simulink model "MultiLoop_mode3"  (Simulink 10.0)
settings: Solver=ode45  StartTime=0.0  StopTime=72  FixedStep=Ts_base  MinStep=1e-6  RelTol=1e-6
values from neighbouring files (symbols this model uses):
  xInitial = xFinal    [prepNextSimIteration.m]
undefined symbols (not defined in the file or in its folder): IDV_Init, r1_0, r4_0, seed, Ts_base, Ts_save
undefined symbols (not defined in the file): SetPoint_Init, SP_deltaTRamp
libraries: TElib x17, simulink x12
settings Model: Creator=ricker  LastModifiedBy=christopher
settings DataIOCC: LoadInitialState=on  SaveFinalState=on  SaveFormat=Structure  SignalLoggingSaveFormat=ModelDataLogs  SaveOutput=off  SaveTime=off  SignalLoggingName=sigsOut
settings OptimizationCC: InitFltsAndDblsToZero=on
settings DebuggingCC: SaveWithParameterizedLinksMsg=none  SignalResolutionControl=TryResolveAllWithWarning  MultiTaskDSMMsg=warning  MultiTaskCondExecSysMsg=none  FcnCallInpInsideContextMsg=warning
settings HardwareCC: TargetUnknown=on
settings GRTTargetCC: TargetFcnLib=ansi_tfl_tmw.mat  GeneratePreprocessorConditionals=Disable all
settings ConfigComp: CovExternalEMLEnable=off  CovSFcnEnable=off

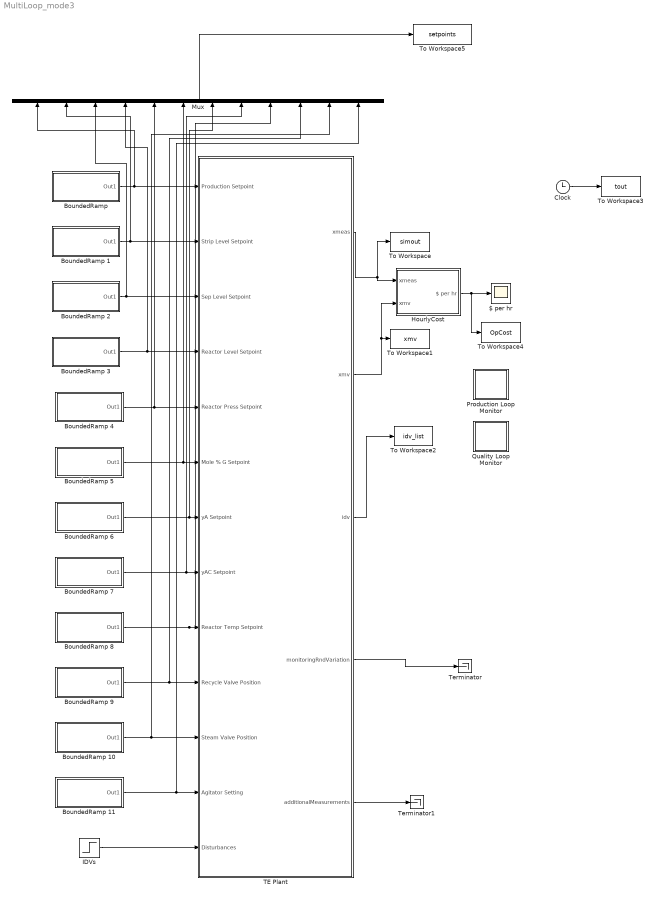
== system MultiLoop_mode3 ==
  $ per hr : Scope
  "BoundedRamp " : Subsystem  mask{SP_before=SetPoint_Init(1,1), SP_after=SetPoint_Init(2,1), tRampStart=SetPoint_Init(3,1), deltaT_ramp=SP_deltaTRamp}
      mask prompts: SP_before "Value before ramp"; SP_after "Value after ramp"; tRampStart "Ramp start time"; deltaT_ramp "Ramp transition time"
  BoundedRamp 1 : Subsystem  mask{SP_before=SetPoint_Init(1,2), SP_after=SetPoint_Init(2,2), tRampStart=SetPoint_Init(3,2), deltaT_ramp=SP_deltaTRamp}
      mask prompts: SP_before "Value before ramp"; SP_after "Value after ramp"; tRampStart "Ramp start time"; deltaT_ramp "Ramp transition time"
  BoundedRamp 10 : Subsystem  mask{SP_before=SetPoint_Init(1,11), SP_after=SetPoint_Init(2,11), tRampStart=SetPoint_Init(3,11), deltaT_ramp=SP_deltaTRamp}
      mask prompts: SP_before "Value before ramp"; SP_after "Value after ramp"; tRampStart "Ramp start time"; deltaT_ramp "Ramp transition time"
  BoundedRamp 11 : Subsystem  mask{SP_before=SetPoint_Init(1,12), SP_after=SetPoint_Init(2,12), tRampStart=SetPoint_Init(3,12), deltaT_ramp=SP_deltaTRamp}
      mask prompts: SP_before "Value before ramp"; SP_after "Value after ramp"; tRampStart "Ramp start time"; deltaT_ramp "Ramp transition time"
  BoundedRamp 2 : Subsystem  mask{SP_before=SetPoint_Init(1,3), SP_after=SetPoint_Init(2,3), tRampStart=SetPoint_Init(3,3), deltaT_ramp=SP_deltaTRamp}
      mask prompts: SP_before "Value before ramp"; SP_after "Value after ramp"; tRampStart "Ramp start time"; deltaT_ramp "Ramp transition time"
  BoundedRamp 3 : Subsystem  mask{SP_before=SetPoint_Init(1,4), SP_after=SetPoint_Init(2,4), tRampStart=SetPoint_Init(3,4), deltaT_ramp=SP_deltaTRamp}
      mask prompts: SP_before "Value before ramp"; SP_after "Value after ramp"; tRampStart "Ramp start time"; deltaT_ramp "Ramp transition time"
  BoundedRamp 4 : Subsystem  mask{SP_before=SetPoint_Init(1,5), SP_after=SetPoint_Init(2,5), tRampStart=SetPoint_Init(3,5), deltaT_ramp=SP_deltaTRamp}
      mask prompts: SP_before "Value before ramp"; SP_after "Value after ramp"; tRampStart "Ramp start time"; deltaT_ramp "Ramp transition time"
  BoundedRamp 5 : Subsystem  mask{SP_before=SetPoint_Init(1,6), SP_after=SetPoint_Init(2,6), tRampStart=SetPoint_Init(3,6), deltaT_ramp=SP_deltaTRamp}
      mask prompts: SP_before "Value before ramp"; SP_after "Value after ramp"; tRampStart "Ramp start time"; deltaT_ramp "Ramp transition time"
  BoundedRamp 6 : Subsystem  mask{SP_before=SetPoint_Init(1,7), SP_after=SetPoint_Init(2,7), tRampStart=SetPoint_Init(3,7), deltaT_ramp=SP_deltaTRamp}
      mask prompts: SP_before "Value before ramp"; SP_after "Value after ramp"; tRampStart "Ramp start time"; deltaT_ramp "Ramp transition time"
  BoundedRamp 7 : Subsystem  mask{SP_before=SetPoint_Init(1,8), SP_after=SetPoint_Init(2,8), tRampStart=SetPoint_Init(3,8), deltaT_ramp=SP_deltaTRamp}
      mask prompts: SP_before "Value before ramp"; SP_after "Value after ramp"; tRampStart "Ramp start time"; deltaT_ramp "Ramp transition time"
  BoundedRamp 8 : Subsystem  mask{SP_before=SetPoint_Init(1,9), SP_after=SetPoint_Init(2,9), tRampStart=SetPoint_Init(3,9), deltaT_ramp=SP_deltaTRamp}
      mask prompts: SP_before "Value before ramp"; SP_after "Value after ramp"; tRampStart "Ramp start time"; deltaT_ramp "Ramp transition time"
  BoundedRamp 9 : Subsystem  mask{SP_before=SetPoint_Init(1,10), SP_after=SetPoint_Init(2,10), tRampStart=SetPoint_Init(3,10), deltaT_ramp=SP_deltaTRamp}
      mask prompts: SP_before "Value before ramp"; SP_after "Value after ramp"; tRampStart "Ramp start time"; deltaT_ramp "Ramp transition time"
  Clock : Clock
  HourlyCost : Subsystem
  IDVs : Step  Time=IDV_Init(3,:)  Before=IDV_Init(1,:)  After=IDV_Init(2,:)  SampleTime=0
  Mux : Mux  Inputs=12
  Production Loop Monitor : Subsystem
  Quality Loop Monitor : Subsystem
  TE Plant : Subsystem
  Terminator : Terminator
  Terminator1 : Terminator
  To Workspace : ToWorkspace  VariableName=simout  SampleTime=Ts_save
  To Workspace1 : ToWorkspace  VariableName=xmv  SampleTime=Ts_save
  To Workspace2 : ToWorkspace  VariableName=idv_list  SampleTime=Ts_save
  To Workspace3 : ToWorkspace  VariableName=tout  SampleTime=Ts_save
  To Workspace4 : ToWorkspace  VariableName=OpCost  SampleTime=Ts_save
  To Workspace5 : ToWorkspace  VariableName=setpoints  SampleTime=Ts_save
  wires:
  TE Plant/1(xmeas) -> HourlyCost/1(xmeas), To Workspace/1
  TE Plant/2(xmv) -> To Workspace1/1, HourlyCost/2(xmv)
  TE Plant/3(idv) -> To Workspace2/1
  Clock/1 -> To Workspace3/1
  HourlyCost/1($ per hr) -> $ per hr/1, To Workspace4/1
  "BoundedRamp "/1(Out1) -> TE Plant/1(Production Setpoint), Mux/1
  BoundedRamp 11/1(Out1) -> Mux/12, TE Plant/12(Agitator Setting)
  BoundedRamp 10/1(Out1) -> Mux/11, TE Plant/11(Steam Valve Position)
  BoundedRamp 9/1(Out1) -> Mux/10, TE Plant/10(Recycle Valve Position)
  BoundedRamp 8/1(Out1) -> Mux/9, TE Plant/9(Reactor Temp Setpoint)
  BoundedRamp 7/1(Out1) -> Mux/8, TE Plant/8(yAC Setpoint)
  BoundedRamp 6/1(Out1) -> Mux/7, TE Plant/7(yA Setpoint)
  BoundedRamp 5/1(Out1) -> Mux/6, TE Plant/6(Mole % G Setpoint)
  BoundedRamp 4/1(Out1) -> TE Plant/5(Reactor Press Setpoint), Mux/5
  BoundedRamp 3/1(Out1) -> TE Plant/4(Reactor Level Setpoint), Mux/4
  BoundedRamp 2/1(Out1) -> TE Plant/3(Sep Level Setpoint), Mux/3
  BoundedRamp 1/1(Out1) -> TE Plant/2(Strip Level Setpoint), Mux/2
  IDVs/1 -> TE Plant/13(Disturbances)
  Mux/1 -> To Workspace5/1
  TE Plant/4(monitoringRndVariation) -> Terminator/1
  TE Plant/5(additionalMeasurements) -> Terminator1/1

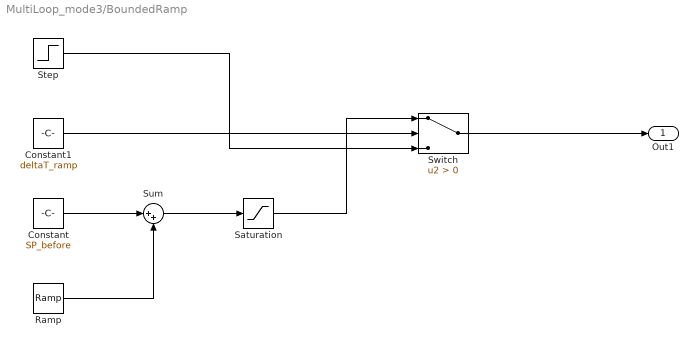
== system MultiLoop_mode3/BoundedRamp  ==
  Constant : Constant  Value=SP_before
  Constant1 : Constant  Value=deltaT_ramp
  Ramp : simulink/Sources/Ramp  slope=(SP_after-SP_before) /max(deltaT_ramp,0.1)  start=tRampStart  InitialOutput=0
  Saturation : Saturate  UpperLimit=max(SP_before, SP_after)  LowerLimit=min(SP_before, SP_after)
  Step : Step  Time=tRampStart  Before=SP_before  After=SP_after  SampleTime=0
  Sum : Sum  Inputs=|++
  Switch : Switch  Criteria=u2 > Threshold
  Out1 : Outport  VectorParamsAs1DForOutWhenUnconnected=off
  wires:
  Constant/1 -> Sum/1
  Ramp/1 -> Sum/2
  Sum/1 -> Saturation/1
  Constant1/1 -> Switch/2
  Switch/1 -> Out1/1
  Step/1 -> Switch/3
  Saturation/1 -> Switch/1

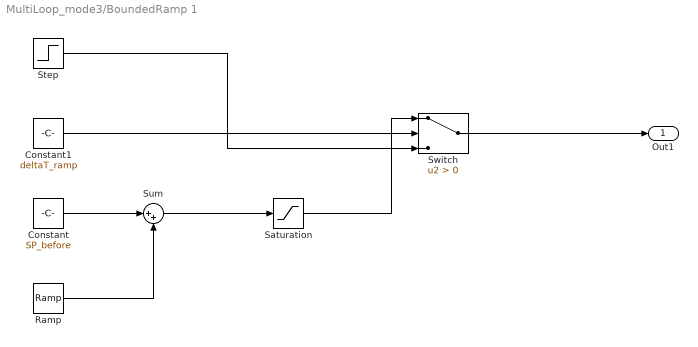
== system MultiLoop_mode3/BoundedRamp 1 ==
  Constant : Constant  Value=SP_before
  Constant1 : Constant  Value=deltaT_ramp
  Ramp : simulink/Sources/Ramp  slope=(SP_after-SP_before) /max(deltaT_ramp,0.1)  start=tRampStart  InitialOutput=0
  Saturation : Saturate  UpperLimit=max(SP_before, SP_after)  LowerLimit=min(SP_before, SP_after)
  Step : Step  Time=tRampStart  Before=SP_before  After=SP_after  SampleTime=0
  Sum : Sum  Inputs=|++
  Switch : Switch  Criteria=u2 > Threshold
  Out1 : Outport  VectorParamsAs1DForOutWhenUnconnected=off
  wires:
  Constant/1 -> Sum/1
  Ramp/1 -> Sum/2
  Sum/1 -> Saturation/1
  Constant1/1 -> Switch/2
  Switch/1 -> Out1/1
  Step/1 -> Switch/3
  Saturation/1 -> Switch/1

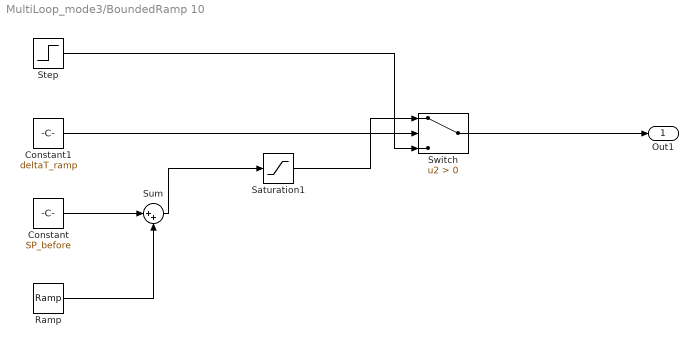
== system MultiLoop_mode3/BoundedRamp 10 ==
  Constant : Constant  Value=SP_before
  Constant1 : Constant  Value=deltaT_ramp
  Ramp : simulink/Sources/Ramp  slope=(SP_after-SP_before) /max(deltaT_ramp,0.1)  start=tRampStart  InitialOutput=0
  Saturation1 : Saturate  UpperLimit=max(SP_before, SP_after)  LowerLimit=min(SP_before, SP_after)
  Step : Step  Time=tRampStart  Before=SP_before  After=SP_after  SampleTime=0
  Sum : Sum  Inputs=|++
  Switch : Switch  Criteria=u2 > Threshold
  Out1 : Outport  VectorParamsAs1DForOutWhenUnconnected=off
  wires:
  Constant/1 -> Sum/1
  Ramp/1 -> Sum/2
  Sum/1 -> Saturation1/1
  Constant1/1 -> Switch/2
  Switch/1 -> Out1/1
  Step/1 -> Switch/3
  Saturation1/1 -> Switch/1

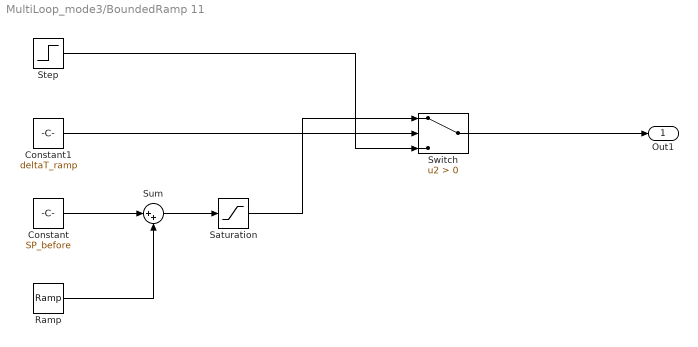
== system MultiLoop_mode3/BoundedRamp 11 ==
  Constant : Constant  Value=SP_before
  Constant1 : Constant  Value=deltaT_ramp
  Ramp : simulink/Sources/Ramp  slope=(SP_after-SP_before) /max(deltaT_ramp,0.1)  start=tRampStart  InitialOutput=0
  Saturation : Saturate  UpperLimit=max(SP_before, SP_after)  LowerLimit=min(SP_before, SP_after)
  Step : Step  Time=tRampStart  Before=SP_before  After=SP_after  SampleTime=0
  Sum : Sum  Inputs=|++
  Switch : Switch  Criteria=u2 > Threshold
  Out1 : Outport  VectorParamsAs1DForOutWhenUnconnected=off
  wires:
  Constant/1 -> Sum/1
  Ramp/1 -> Sum/2
  Sum/1 -> Saturation/1
  Constant1/1 -> Switch/2
  Switch/1 -> Out1/1
  Step/1 -> Switch/3
  Saturation/1 -> Switch/1

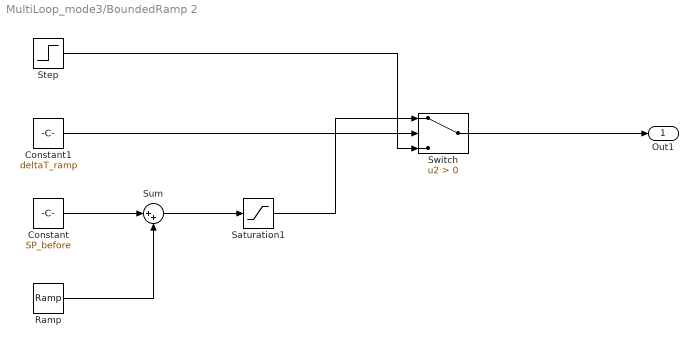
== system MultiLoop_mode3/BoundedRamp 2 ==
  Constant : Constant  Value=SP_before
  Constant1 : Constant  Value=deltaT_ramp
  Ramp : simulink/Sources/Ramp  slope=(SP_after-SP_before) /max(deltaT_ramp,0.1)  start=tRampStart  InitialOutput=0
  Saturation1 : Saturate  UpperLimit=max(SP_before, SP_after)  LowerLimit=min(SP_before, SP_after)
  Step : Step  Time=tRampStart  Before=SP_before  After=SP_after  SampleTime=0
  Sum : Sum  Inputs=|++
  Switch : Switch  Criteria=u2 > Threshold
  Out1 : Outport  VectorParamsAs1DForOutWhenUnconnected=off
  wires:
  Constant/1 -> Sum/1
  Ramp/1 -> Sum/2
  Sum/1 -> Saturation1/1
  Constant1/1 -> Switch/2
  Switch/1 -> Out1/1
  Step/1 -> Switch/3
  Saturation1/1 -> Switch/1

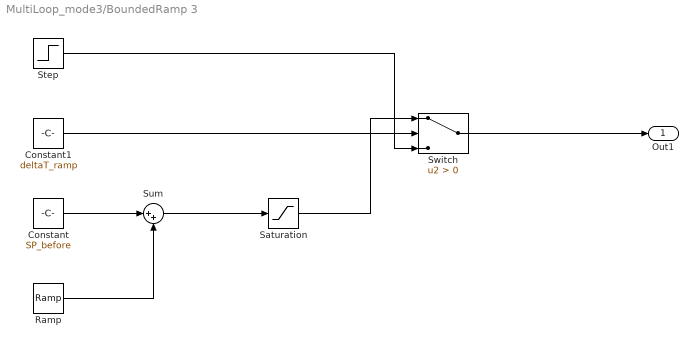
== system MultiLoop_mode3/BoundedRamp 3 ==
  Constant : Constant  Value=SP_before
  Constant1 : Constant  Value=deltaT_ramp
  Ramp : simulink/Sources/Ramp  slope=(SP_after-SP_before) /max(deltaT_ramp,0.1)  start=tRampStart  InitialOutput=0
  Saturation : Saturate  UpperLimit=max(SP_before, SP_after)  LowerLimit=min(SP_before, SP_after)
  Step : Step  Time=tRampStart  Before=SP_before  After=SP_after  SampleTime=0
  Sum : Sum  Inputs=|++
  Switch : Switch  Criteria=u2 > Threshold
  Out1 : Outport  VectorParamsAs1DForOutWhenUnconnected=off
  wires:
  Constant/1 -> Sum/1
  Ramp/1 -> Sum/2
  Sum/1 -> Saturation/1
  Constant1/1 -> Switch/2
  Switch/1 -> Out1/1
  Step/1 -> Switch/3
  Saturation/1 -> Switch/1

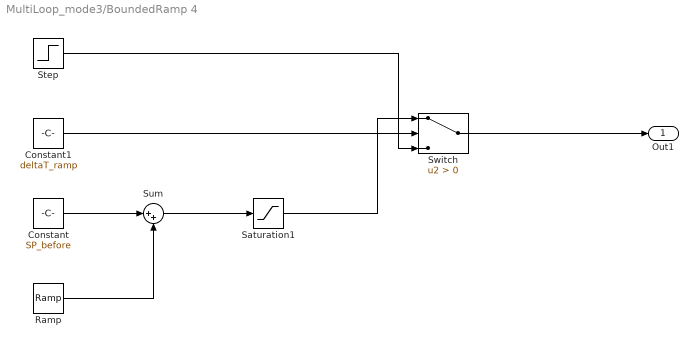
== system MultiLoop_mode3/BoundedRamp 4 ==
  Constant : Constant  Value=SP_before
  Constant1 : Constant  Value=deltaT_ramp
  Ramp : simulink/Sources/Ramp  slope=(SP_after-SP_before) /max(deltaT_ramp,0.1)  start=tRampStart  InitialOutput=0
  Saturation1 : Saturate  UpperLimit=max(SP_before, SP_after)  LowerLimit=min(SP_before, SP_after)
  Step : Step  Time=tRampStart  Before=SP_before  After=SP_after  SampleTime=0
  Sum : Sum  Inputs=|++
  Switch : Switch  Criteria=u2 > Threshold
  Out1 : Outport  VectorParamsAs1DForOutWhenUnconnected=off
  wires:
  Constant/1 -> Sum/1
  Ramp/1 -> Sum/2
  Sum/1 -> Saturation1/1
  Constant1/1 -> Switch/2
  Switch/1 -> Out1/1
  Step/1 -> Switch/3
  Saturation1/1 -> Switch/1

== system MultiLoop_mode3/BoundedRamp 5 ==
  Constant : Constant  Value=SP_before
  Constant1 : Constant  Value=deltaT_ramp
  Ramp : simulink/Sources/Ramp  slope=(SP_after-SP_before) /max(deltaT_ramp,0.1)  start=tRampStart  InitialOutput=0
  Saturation1 : Saturate  UpperLimit=max(SP_before, SP_after)  LowerLimit=min(SP_before, SP_after)
  Step : Step  Time=tRampStart  Before=SP_before  After=SP_after  SampleTime=0
  Sum : Sum  Inputs=|++
  Switch : Switch  Criteria=u2 > Threshold
  Out1 : Outport  VectorParamsAs1DForOutWhenUnconnected=off
  wires:
  Constant/1 -> Sum/1
  Ramp/1 -> Sum/2
  Sum/1 -> Saturation1/1
  Constant1/1 -> Switch/2
  Switch/1 -> Out1/1
  Step/1 -> Switch/3
  Saturation1/1 -> Switch/1

== system MultiLoop_mode3/BoundedRamp 6 ==
  Constant : Constant  Value=SP_before
  Constant1 : Constant  Value=deltaT_ramp
  Ramp : simulink/Sources/Ramp  slope=(SP_after-SP_before) /max(deltaT_ramp,0.1)  start=tRampStart  InitialOutput=0
  Saturation1 : Saturate  UpperLimit=max(SP_before, SP_after)  LowerLimit=min(SP_before, SP_after)
  Step : Step  Time=tRampStart  Before=SP_before  After=SP_after  SampleTime=0
  Sum : Sum  Inputs=|++
  Switch : Switch  Criteria=u2 > Threshold
  Out1 : Outport  VectorParamsAs1DForOutWhenUnconnected=off
  wires:
  Constant/1 -> Sum/1
  Ramp/1 -> Sum/2
  Sum/1 -> Saturation1/1
  Constant1/1 -> Switch/2
  Switch/1 -> Out1/1
  Step/1 -> Switch/3
  Saturation1/1 -> Switch/1

== system MultiLoop_mode3/BoundedRamp 7 ==
  Constant : Constant  Value=SP_before
  Constant1 : Constant  Value=deltaT_ramp
  Ramp : simulink/Sources/Ramp  slope=(SP_after-SP_before) /max(deltaT_ramp,0.1)  start=tRampStart  InitialOutput=0
  Saturation1 : Saturate  UpperLimit=max(SP_before, SP_after)  LowerLimit=min(SP_before, SP_after)
  Step : Step  Time=tRampStart  Before=SP_before  After=SP_after  SampleTime=0
  Sum : Sum  Inputs=|++
  Switch : Switch  Criteria=u2 > Threshold
  Out1 : Outport  VectorParamsAs1DForOutWhenUnconnected=off
  wires:
  Constant/1 -> Sum/1
  Ramp/1 -> Sum/2
  Sum/1 -> Saturation1/1
  Constant1/1 -> Switch/2
  Switch/1 -> Out1/1
  Step/1 -> Switch/3
  Saturation1/1 -> Switch/1

== system MultiLoop_mode3/BoundedRamp 8 ==
  Constant : Constant  Value=SP_before
  Constant1 : Constant  Value=deltaT_ramp
  Ramp : simulink/Sources/Ramp  slope=(SP_after-SP_before) /max(deltaT_ramp,0.1)  start=tRampStart  InitialOutput=0
  Saturation1 : Saturate  UpperLimit=max(SP_before, SP_after)  LowerLimit=min(SP_before, SP_after)
  Step : Step  Time=tRampStart  Before=SP_before  After=SP_after  SampleTime=0
  Sum : Sum  Inputs=|++
  Switch : Switch  Criteria=u2 > Threshold
  Out1 : Outport  VectorParamsAs1DForOutWhenUnconnected=off
  wires:
  Constant/1 -> Sum/1
  Ramp/1 -> Sum/2
  Sum/1 -> Saturation1/1
  Constant1/1 -> Switch/2
  Switch/1 -> Out1/1
  Step/1 -> Switch/3
  Saturation1/1 -> Switch/1

== system MultiLoop_mode3/BoundedRamp 9 ==
  Constant : Constant  Value=SP_before
  Constant1 : Constant  Value=deltaT_ramp
  Ramp : simulink/Sources/Ramp  slope=(SP_after-SP_before) /max(deltaT_ramp,0.1)  start=tRampStart  InitialOutput=0
  Saturation1 : Saturate  UpperLimit=max(SP_before, SP_after)  LowerLimit=min(SP_before, SP_after)
  Step : Step  Time=tRampStart  Before=SP_before  After=SP_after  SampleTime=0
  Sum : Sum  Inputs=|++
  Switch : Switch  Criteria=u2 > Threshold
  Out1 : Outport  VectorParamsAs1DForOutWhenUnconnected=off
  wires:
  Constant/1 -> Sum/1
  Ramp/1 -> Sum/2
  Sum/1 -> Saturation1/1
  Constant1/1 -> Switch/2
  Switch/1 -> Out1/1
  Step/1 -> Switch/3
  Saturation1/1 -> Switch/1

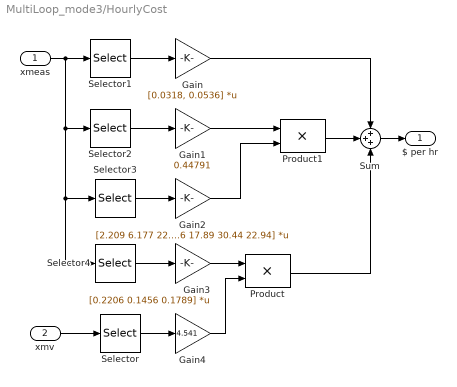
== system MultiLoop_mode3/HourlyCost ==
  xmeas : Inport  PortDimensions=41
  xmv : Inport  Port=2  PortDimensions=12
  Gain : Gain  Gain=[0.0318, 0.0536]  Multiplication=Matrix(K*u)  SaturateOnIntegerOverflow=on  OutDataTypeStr=Inherit: Same as input  ParamDataTypeStr=Inherit: Same as input
  Gain1 : Gain  Gain=0.44791  SaturateOnIntegerOverflow=on  OutDataTypeStr=Inherit: Same as input  ParamDataTypeStr=Inherit: Same as input
  Gain2 : Gain  Gain=[2.209 6.177 22.06 14.56 17.89 30.44 22.94]  Multiplication=Matrix(K*u)  SaturateOnIntegerOverflow=on  OutDataTypeStr=Inherit: Same as input  ParamDataTypeStr=Inherit: Same as input
  Gain3 : Gain  Gain=[0.2206 0.1456 0.1789]  Multiplication=Matrix(K*u)  SaturateOnIntegerOverflow=on  OutDataTypeStr=Inherit: Same as input  ParamDataTypeStr=Inherit: Same as input
  Gain4 : Gain  Gain=4.541  SaturateOnIntegerOverflow=on  OutDataTypeStr=Inherit: Same as input  ParamDataTypeStr=Inherit: Same as input
  Product : Product  SaturateOnIntegerOverflow=on  OutDataTypeStr=Inherit: Same as first input
  Product1 : Product  SaturateOnIntegerOverflow=on  OutDataTypeStr=Inherit: Same as first input
  Selector : Selector  InputPortWidth=12  IndexOptions=Index vector (dialog)  Indices=8  OutputSizes=1
  Selector1 : Selector  InputPortWidth=41  IndexOptions=Index vector (dialog)  Indices=[19 20]  OutputSizes=1
  Selector2 : Selector  InputPortWidth=41  IndexOptions=Index vector (dialog)  Indices=[10]  OutputSizes=1
  Selector3 : Selector  InputPortWidth=41  IndexOptions=Index vector (dialog)  Indices=[29, 31:36]  OutputSizes=1
  Selector4 : Selector  InputPortWidth=41  IndexOptions=Index vector (dialog)  Indices=[37:39]  OutputSizes=1
  Sum : Sum  Inputs=+++  SaturateOnIntegerOverflow=on
  $ per hr : Outport  VectorParamsAs1DForOutWhenUnconnected=off
  wires:
  xmv/1 -> Selector/1
  xmeas/1 -> Selector1/1, Selector2/1, Selector3/1, Selector4/1
  Selector1/1 -> Gain/1
  Selector2/1 -> Gain1/1
  Selector3/1 -> Gain2/1
  Selector4/1 -> Gain3/1
  Selector/1 -> Gain4/1
  Gain3/1 -> Product/1
  Gain4/1 -> Product/2
  Sum/1 -> $ per hr/1
  Product/1 -> Sum/3
  Gain/1 -> Sum/1
  Product1/1 -> Sum/2
  Gain1/1 -> Product1/1
  Gain2/1 -> Product1/2

== system MultiLoop_mode3/Production Loop Monitor ==
  Mux2 : Mux  Inputs=2
  Production : Scope
  wires:
  Mux2/1 -> Production/1
  [xmeas17] -> Mux2/2
  [Prodsp] -> Mux2/1

== system MultiLoop_mode3/Quality Loop Monitor ==
  Mux2 : Mux  Inputs=2
  Quality : Scope
  wires:
  [PctGsp] -> Mux2/1
  [xmeas40] -> Mux2/2
  Mux2/1 -> Quality/1

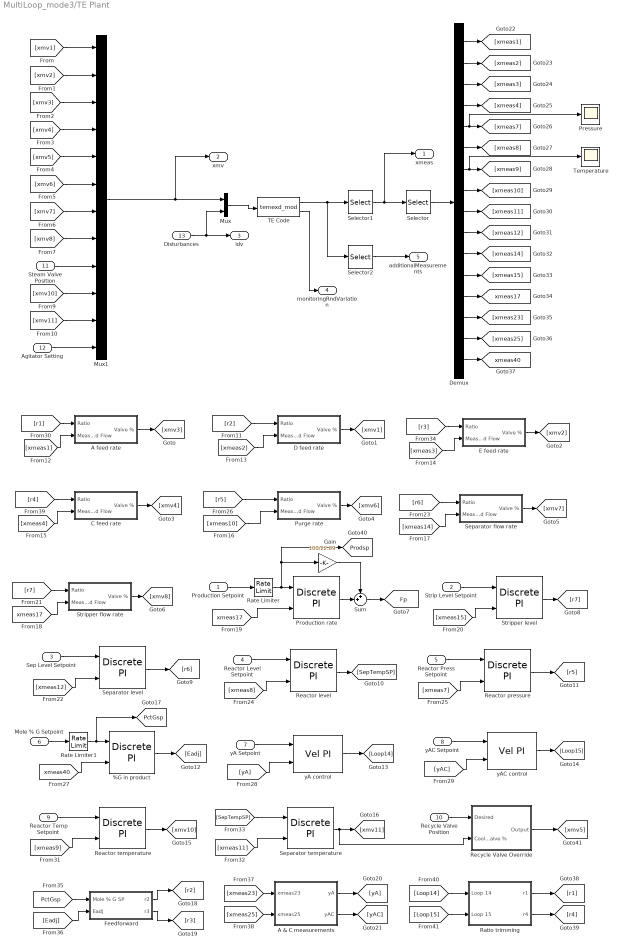
== system MultiLoop_mode3/TE Plant ==
  Production Setpoint : Inport
  Strip Level Setpoint : Inport  Port=2
  Sep Level Setpoint : Inport  Port=3
  Reactor Level Setpoint : Inport  Port=4
  Reactor Press Setpoint : Inport  Port=5
  Mole % G Setpoint : Inport  Port=6
  yA Setpoint : Inport  Port=7
  yAC Setpoint : Inport  Port=8
  Reactor Temp Setpoint : Inport  Port=9
  Recycle Valve Position : Inport  Port=10
  Steam Valve Position : Inport  Port=11
  Agitator Setting : Inport  Port=12
  Disturbances : Inport  Port=13
  %G in product : TElib/Discrete PI  Kc=-0.4  Ti=100/60  Ts=Ts_base  x0=Eadj_0  Hi=inf  Lo=-inf
  A & C measurements : Subsystem
  A feed rate : Subsystem
  C feed rate : Subsystem
  D feed rate : Subsystem
  Demux : Demux  Outputs=16
  E feed rate : Subsystem
  Feedforward : Subsystem
  Gain : Gain  Gain=100/22.89  SaturateOnIntegerOverflow=on  OutDataTypeStr=Inherit: Same as input  ParamDataTypeStr=Inherit: Same as input
  Mux : Mux  Inputs=2
  Mux1 : Mux  Inputs=12
  Pressure : Scope
  Production rate : TElib/Discrete PI  Kc=3.2  Ti=120/60  Ts=Ts_base  x0=0  Hi=30  Lo=-30
  Purge rate : Subsystem
  Rate Limiter : RateLimiter  RisingSlewLimit=0.3*22.95/24  FallingSlewLimit=-0.3*22.95/24
  Rate Limiter1 : RateLimiter  RisingSlewLimit=50/24  FallingSlewLimit=-50/24
  Ratio trimming : Subsystem
  Reactor level : TElib/Discrete PI  Kc=0.8  Ti=60/60  Ts=Ts_base  x0=SP17_0  Hi=120  Lo=0
  Reactor pressure : TElib/Discrete PI  Kc=-1e-4  Ti=20/60  Ts=Ts_base  x0=r5_0  Hi=100  Lo=0
  Reactor temperature : TElib/Discrete PI  Kc=-8  Ti=7.5/60  Ts=Ts_base  x0=xmv10_0  Hi=100  Lo=0
  Recycle Valve Override : Subsystem  AncestorBlock=TElib/Discrete PI
  Selector : Selector  InputPortWidth=41  IndexOptions=Index vector (dialog)  Indices=[1:4, 7:12, 14, 15, 17, 23, 25, 40]  OutputSizes=1
  Selector1 : Selector  InputPortWidth=73  IndexOptions=Index vector (dialog)  Indices=[1:41]  OutputSizes=1
  Selector2 : Selector  InputPortWidth=73  IndexOptions=Index vector (dialog)  Indices=[42:73]  OutputSizes=1
  Separator flow rate : Subsystem
  Separator level : TElib/Discrete PI  Kc=-1e-3  Ti=200/60  Ts=Ts_base  x0=r6_0  Hi=100  Lo=0
  Separator temperature : TElib/Discrete PI  Kc=-4  Ti=15/60  Ts=Ts_base  x0=xmv11_0  Hi=100  Lo=0
  Stripper flow rate : Subsystem
  Stripper level : TElib/Discrete PI  Kc=-2e-4  Ti=200/60  Ts=Ts_base  x0=r7_0  Hi=100  Lo=0
  Sum : Sum  Inputs=++|  SaturateOnIntegerOverflow=on
  TE Code : S-Function  FunctionName=temexd_mod  Parameters=xInitial.signals(1).values,seed,243  SFunctionDeploymentMode=off  EnableBusSupport=off
  Temperature : Scope
  yA control : TElib/Discrete PI/Vel PI  Kc=2e-4  Ti=1  Ts=0.1
  yAC control : TElib/Discrete PI/Vel PI  Kc=3e-4  Ti=2  Ts=0.1
  xmeas : Outport  VectorParamsAs1DForOutWhenUnconnected=off
  xmv : Outport  Port=2  VectorParamsAs1DForOutWhenUnconnected=off
  idv : Outport  Port=3  VectorParamsAs1DForOutWhenUnconnected=off
  monitoringRndVariation : Outport  Port=4  VectorParamsAs1DForOutWhenUnconnected=off
  additionalMeasurements : Outport  Port=5  VectorParamsAs1DForOutWhenUnconnected=off
  tag scope: Fp=global, PctGsp=global, Prodsp=global, xmeas17=global, xmeas40=global
  wires:
  Mux/1 -> TE Code/1
  Disturbances/1 -> Mux/2, idv/1
  TE Code/1 -> Selector2/1, Selector1/1
  [xmv1] -> Mux1/1
  [xmv2] -> Mux1/2
  [xmv3] -> Mux1/3
  [xmv4] -> Mux1/4
  [xmv6] -> Mux1/6
  [xmv7] -> Mux1/7
  [xmv8] -> Mux1/8
  Steam Valve Position/1 -> Mux1/9
  [xmv10] -> Mux1/10
  [xmv11] -> Mux1/11
  Agitator Setting/1 -> Mux1/12
  A feed rate/1(Valve %) -> [xmv3]
  [xmeas1] -> A feed rate/2(Measured Flow)
  D feed rate/1(Valve %) -> [xmv1]
  [xmeas2] -> D feed rate/2(Measured Flow)
  E feed rate/1(Valve %) -> [xmv2]
  [xmeas3] -> E feed rate/2(Measured Flow)
  C feed rate/1(Valve %) -> [xmv4]
  [xmeas4] -> C feed rate/2(Measured Flow)
  Purge rate/1(Valve %) -> [xmv6]
  [xmeas10] -> Purge rate/2(Measured Flow)
  Separator flow rate/1(Valve %) -> [xmv7]
  [xmeas14] -> Separator flow rate/2(Measured Flow)
  Stripper flow rate/1(Valve %) -> [xmv8]
  [xmeas17] -> Stripper flow rate/2(Measured Flow)
  [xmeas17] -> Production rate/2
  [xmeas15] -> Stripper level/2
  Strip Level Setpoint/1 -> Stripper level/1
  Stripper level/1 -> [r7]
  [r7] -> Stripper flow rate/1(Ratio)
  [xmeas12] -> Separator level/2
  Sep Level Setpoint/1 -> Separator level/1
  Separator level/1 -> [r6]
  [r6] -> Separator flow rate/1(Ratio)
  [xmeas8] -> Reactor level/2
  Reactor Level Setpoint/1 -> Reactor level/1
  Reactor level/1 -> [SepTempSP]
  [xmeas7] -> Reactor pressure/2
  Reactor Press Setpoint/1 -> Reactor pressure/1
  Reactor pressure/1 -> [r5]
  [r5] -> Purge rate/1(Ratio)
  [xmeas40] -> %G in product/2
  %G in product/1 -> [Eadj]
  [yA] -> yA control/2
  yA Setpoint/1 -> yA control/1
  yA control/1 -> [Loop14]
  [yAC] -> yAC control/2
  yAC Setpoint/1 -> yAC control/1
  yAC control/1 -> [Loop15]
  [r1] -> A feed rate/1(Ratio)
  [xmeas9] -> Reactor temperature/2
  Reactor Temp Setpoint/1 -> Reactor temperature/1
  Reactor temperature/1 -> [xmv10]
  [xmeas11] -> Separator temperature/2
  [SepTempSP] -> Separator temperature/1
  Separator temperature/1 -> [xmv11], Recycle Valve Override/2(Coolant Valve %)
  [r2] -> D feed rate/1(Ratio)
  [r3] -> E feed rate/1(Ratio)
  [PctGsp] -> Feedforward/1(Mole % G SP)
  [Eadj] -> Feedforward/2(Eadj)
  Feedforward/1(r2) -> [r2]
  Feedforward/2(r3) -> [r3]
  [xmeas23] -> A & C measurements/1(xmeas23)
  [xmeas25] -> A & C measurements/2(xmeas25)
  A & C measurements/1(yA) -> [yA]
  A & C measurements/2(yAC) -> [yAC]
  Mux1/1 -> Mux/1, xmv/1
  Selector/1 -> Demux/1
  Demux/1 -> [xmeas1]
  Demux/2 -> [xmeas2]
  Demux/3 -> [xmeas3]
  Demux/4 -> [xmeas4]
  Demux/5 -> [xmeas7], Pressure/1
  Demux/6 -> [xmeas8]
  Demux/7 -> [xmeas9], Temperature/1
  Demux/8 -> [xmeas10]
  Demux/9 -> [xmeas11]
  Demux/10 -> [xmeas12]
  Demux/11 -> [xmeas14]
  Demux/12 -> [xmeas15]
  Demux/13 -> [xmeas17]
  Demux/14 -> [xmeas23]
  Demux/15 -> [xmeas25]
  Demux/16 -> [xmeas40]
  [r4] -> C feed rate/1(Ratio)
  [Loop14] -> Ratio trimming/1(Loop 14)
  [Loop15] -> Ratio trimming/2(Loop 15)
  Ratio trimming/1(r1) -> [r1]
  Ratio trimming/2(r4) -> [r4]
  Production Setpoint/1 -> Rate Limiter/1
  Rate Limiter/1 -> Production rate/1, [Prodsp], Gain/1
  Mole % G Setpoint/1 -> Rate Limiter1/1
  Rate Limiter1/1 -> %G in product/1, [PctGsp]
  Production rate/1 -> Sum/2
  Sum/1 -> [Fp]
  Gain/1 -> Sum/1
  [xmv5] -> Mux1/5
  Recycle Valve Override/1(Output) -> [xmv5]
  Recycle Valve Position/1 -> Recycle Valve Override/1(Desired)
  Selector2/1 -> additionalMeasurements/1
  TE Code/2 -> monitoringRndVariation/1
  Selector1/1 -> xmeas/1, Selector/1

== system MultiLoop_mode3/TE Plant/A & C measurements ==
  xmeas23 : Inport
  xmeas25 : Inport  Port=2
  Gain1 : Gain  Gain=100  SaturateOnIntegerOverflow=on  OutDataTypeStr=Inherit: Same as input  ParamDataTypeStr=Inherit: Same as input
  Product1 : Product  Inputs=*/  SaturateOnIntegerOverflow=on  OutDataTypeStr=Inherit: Same as first input
  Sum1 : Sum  Inputs=++|  SaturateOnIntegerOverflow=on
  yA : Outport  VectorParamsAs1DForOutWhenUnconnected=off
  yAC : Outport  Port=2  VectorParamsAs1DForOutWhenUnconnected=off
  wires:
  Sum1/1 -> yAC/1, Product1/2
  xmeas23/1 -> Sum1/1, Gain1/1
  xmeas25/1 -> Sum1/2
  Gain1/1 -> Product1/1
  Product1/1 -> yA/1

== system MultiLoop_mode3/TE Plant/A feed rate ==
  Ratio : Inport
  Measured Flow : Inport  Port=2
  Discrete PI : TElib/Discrete PI  Kc=0.01  Ti=0.001/60  Ts=Ts_base  x0=xmv3_0  Hi=100  Lo=0
  Product : Product  SaturateOnIntegerOverflow=on  OutDataTypeStr=Inherit: Same as first input
  Valve % : Outport  VectorParamsAs1DForOutWhenUnconnected=off
  wires:
  Discrete PI/1 -> Valve %/1
  Ratio/1 -> Product/1
  [Fp] -> Product/2
  Measured Flow/1 -> Discrete PI/2
  Product/1 -> Discrete PI/1

== system MultiLoop_mode3/TE Plant/C feed rate ==
  Ratio : Inport
  Measured Flow : Inport  Port=2
  Discrete PI : TElib/Discrete PI  Kc=0.003  Ti=0.001/60  Ts=Ts_base  x0=xmv4_0  Hi=100  Lo=0
  Product : Product  SaturateOnIntegerOverflow=on  OutDataTypeStr=Inherit: Same as first input
  Valve % : Outport  VectorParamsAs1DForOutWhenUnconnected=off
  wires:
  Product/1 -> Discrete PI/1
  Measured Flow/1 -> Discrete PI/2
  [Fp] -> Product/2
  Ratio/1 -> Product/1
  Discrete PI/1 -> Valve %/1

== system MultiLoop_mode3/TE Plant/D feed rate ==
  Ratio : Inport
  Measured Flow : Inport  Port=2
  Discrete PI : TElib/Discrete PI  Kc=1.6e-6  Ti=0.001/60  Ts=Ts_base  x0=xmv1_0  Hi=100  Lo=0
  Product : Product  SaturateOnIntegerOverflow=on  OutDataTypeStr=Inherit: Same as first input
  Valve % : Outport  VectorParamsAs1DForOutWhenUnconnected=off
  wires:
  Product/1 -> Discrete PI/1
  Measured Flow/1 -> Discrete PI/2
  [Fp] -> Product/2
  Ratio/1 -> Product/1
  Discrete PI/1 -> Valve %/1

== system MultiLoop_mode3/TE Plant/E feed rate ==
  Ratio : Inport
  Measured Flow : Inport  Port=2
  Discrete PI : TElib/Discrete PI  Kc=1.8e-6  Ti=0.001/60  Ts=Ts_base  x0=xmv2_0  Hi=100  Lo=0
  Product : Product  SaturateOnIntegerOverflow=on  OutDataTypeStr=Inherit: Same as first input
  Valve % : Outport  VectorParamsAs1DForOutWhenUnconnected=off
  wires:
  Product/1 -> Discrete PI/1
  Measured Flow/1 -> Discrete PI/2
  [Fp] -> Product/2
  Ratio/1 -> Product/1
  Discrete PI/1 -> Valve %/1

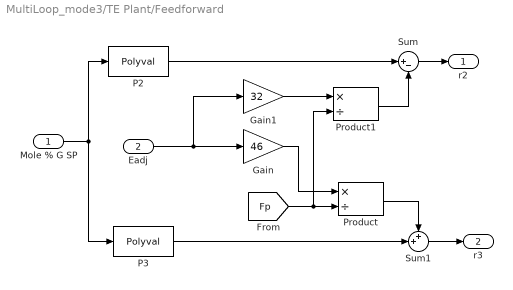
== system MultiLoop_mode3/TE Plant/Feedforward ==
  Mole % G SP : Inport
  Eadj : Inport  Port=2
  Gain : Gain  Gain=46  SaturateOnIntegerOverflow=on  OutDataTypeStr=Inherit: Same as input  ParamDataTypeStr=Inherit: Same as input
  Gain1 : Gain  Gain=32  SaturateOnIntegerOverflow=on  OutDataTypeStr=Inherit: Same as input  ParamDataTypeStr=Inherit: Same as input
  P2 : Polyval  Coefs="[1.5192e-003  5.9446e-001  2.7690e-001]"
  P3 : Polyval  Coefs="[-1.1377e-003 -8.0893e-001  9.1060e+001]"
  Product : Product  Inputs=*/  SaturateOnIntegerOverflow=on  OutDataTypeStr=Inherit: Same as first input
  Product1 : Product  Inputs=*/  SaturateOnIntegerOverflow=on  OutDataTypeStr=Inherit: Same as first input
  Sum : Sum  Inputs=|+-  SaturateOnIntegerOverflow=on
  Sum1 : Sum  Inputs=++|  SaturateOnIntegerOverflow=on
  r2 : Outport  VectorParamsAs1DForOutWhenUnconnected=off
  r3 : Outport  Port=2  VectorParamsAs1DForOutWhenUnconnected=off
  wires:
  Mole % G SP/1 -> P2/1, P3/1
  Sum/1 -> r2/1
  P2/1 -> Sum/1
  Sum1/1 -> r3/1
  P3/1 -> Sum1/2
  Product/1 -> Sum1/1
  [Fp] -> Product/2, Product1/2
  Gain/1 -> Product/1
  Eadj/1 -> Gain/1, Gain1/1
  Product1/1 -> Sum/2
  Gain1/1 -> Product1/1

== system MultiLoop_mode3/TE Plant/Purge rate ==
  Ratio : Inport
  Measured Flow : Inport  Port=2
  Discrete PI : TElib/Discrete PI  Kc=0.01  Ti=0.001/60  Ts=Ts_base  x0=xmv6_0  Hi=100  Lo=0
  Product : Product  SaturateOnIntegerOverflow=on  OutDataTypeStr=Inherit: Same as first input
  Valve % : Outport  VectorParamsAs1DForOutWhenUnconnected=off
  wires:
  Discrete PI/1 -> Valve %/1
  Ratio/1 -> Product/1
  [Fp] -> Product/2
  Measured Flow/1 -> Discrete PI/2
  Product/1 -> Discrete PI/1

== system MultiLoop_mode3/TE Plant/Ratio trimming ==
  Loop 14 : Inport
  Loop 15 : Inport  Port=2
  Sum1 : Sum  Inputs=-++  SaturateOnIntegerOverflow=on
  Sum2 : Sum  Inputs=++|  SaturateOnIntegerOverflow=on
  Unit Delay : UnitDelay  InitialCondition=r1_0  SampleTime=0.1  HasFrameUpgradeWarning=on
  Unit Delay1 : UnitDelay  InitialCondition=r4_0  SampleTime=0.1  HasFrameUpgradeWarning=on
  r1 : Outport  VectorParamsAs1DForOutWhenUnconnected=off
  r4 : Outport  Port=2  VectorParamsAs1DForOutWhenUnconnected=off
  wires:
  Loop 15/1 -> Sum1/2
  Unit Delay/1 -> Sum2/1
  Unit Delay1/1 -> Sum1/3
  Sum2/1 -> Unit Delay/1, r1/1
  Loop 14/1 -> Sum2/2, Sum1/1
  Sum1/1 -> Unit Delay1/1, r4/1

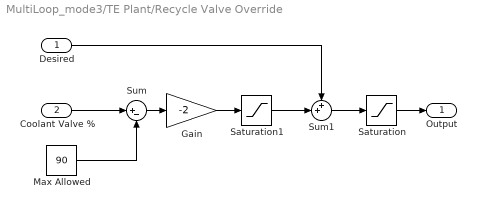
== system MultiLoop_mode3/TE Plant/Recycle Valve Override ==
  Desired : Inport
  Coolant Valve % : Inport  Port=2
  Gain : Gain  Gain=-2
  Max Allowed : Constant  Value=90
  Saturation : Saturate  UpperLimit=100  LowerLimit=0
  Saturation1 : Saturate  UpperLimit=0  LowerLimit=-Inf
  Sum : Sum  Inputs=|+-  SaturateOnIntegerOverflow=on
  Sum1 : Sum  Inputs=++|
  Output : Outport  VectorParamsAs1DForOutWhenUnconnected=off
  wires:
  Saturation/1 -> Output/1
  Coolant Valve %/1 -> Sum/1
  Sum/1 -> Gain/1
  Max Allowed/1 -> Sum/2
  Gain/1 -> Saturation1/1
  Sum1/1 -> Saturation/1
  Saturation1/1 -> Sum1/2
  Desired/1 -> Sum1/1

== system MultiLoop_mode3/TE Plant/Separator flow rate ==
  Ratio : Inport
  Measured Flow : Inport  Port=2
  Discrete PI : TElib/Discrete PI  Kc=4e-4  Ti=0.001/60  Ts=Ts_base  x0=xmv7_0  Hi=100  Lo=0
  Product : Product  SaturateOnIntegerOverflow=on  OutDataTypeStr=Inherit: Same as first input
  Valve % : Outport  VectorParamsAs1DForOutWhenUnconnected=off
  wires:
  Product/1 -> Discrete PI/1
  Measured Flow/1 -> Discrete PI/2
  [Fp] -> Product/2
  Ratio/1 -> Product/1
  Discrete PI/1 -> Valve %/1

== system MultiLoop_mode3/TE Plant/Stripper flow rate ==
  Ratio : Inport
  Measured Flow : Inport  Port=2
  Discrete PI : TElib/Discrete PI  Kc=4e-4  Ti=0.001/60  Ts=Ts_base  x0=xmv8_0  Hi=100  Lo=0
  Product : Product  SaturateOnIntegerOverflow=on  OutDataTypeStr=Inherit: Same as first input
  Valve % : Outport  VectorParamsAs1DForOutWhenUnconnected=off
  wires:
  Discrete PI/1 -> Valve %/1
  Ratio/1 -> Product/1
  [Fp] -> Product/2
  Measured Flow/1 -> Discrete PI/2
  Product/1 -> Discrete PI/1
